simulink model "run_2022"  (R2022b)
settings: Solver=VariableStepAuto  StartTime=t_i  StopTime=2  MaxStep=s_max  RelTol=1e-3
InitFcn:
  | data;
  | init;
values from neighbouring files (symbols this model uses):
  h_ej = 0.15    [data.m]
  phi_0 = atan(-(r_ej*h_0)/(h_ej^2*sqrt(1-h_0^2/h_ej^2)))    [init.m]
  r_0 = sqrt((r_ej^2)*(1-h_0^2/h_ej^2))    [init.m]
  r_ej = 0.0821    [data.m]
  T_d = 1e-20    [data.m]
  x_ej = -0.05    [data.m]
  y_ej = 0.06    [data.m]
  z_ej = -0.03    [data.m]
undefined symbols (not defined in the file or in its folder): Glenohumeral_F0M, Glenohumeral_l0, Scapulothoracic_F0M, Scapulothoracic_l0, X, Y, Z
libraries: sm_lib x148, nesl_utility x62
(part 4 of 4)

== system run_2022/Scapulothoracic/TRP3 ==
  Aktivace : Inport
  Active_factor_norm : MATLAB Function  TreatAsAtomicUnit=on
  F0M : Gain  Gain=Scapulothoracic_F0M(7)
  Internal Force1 : sm_lib/Forces and Torques/Internal Force
  PECM1_3 : sm_lib/Frames and Transforms/Rigid Transform  TranslationMethod=Cartesian  TranslationStandardOffset=0  TranslationStandardOffsetUnits=m  TranslationStandardAxis=+Z  TranslationCartesianOffset=[-0.092 -0.015 0.003]  TranslationCartesianOffsetUnits=m  TranslationROffset=0  TranslationROffsetUnits=m  TranslationZOffset=0  TranslationZOffsetUnits=m  TranslationThetaOffset=0  TranslationThetaOffsetUnits=deg  RotationMethod=None  RotationAngleUnits=deg  RotationStandardAxis=+Z  RotationAngle=0.0  RotationArbitraryAxis=[0 0 1]  FollAlignAxisA=+X  BaseAlignAxisA=+Y  FollAlignAxisB=+Y  BaseAlignAxisB=+Z  RotationSequenceAxes=FollowerAxes  RotationSequence=XYX  RotationSequenceAngles=[0 0 0]  RotationSequenceAnglesUnits=deg  RotationMatrix=[1 0 0; 0 1 0; 0 0 1]  Quaternion=[1 0 0 0]
  PECM1_4 : sm_lib/Frames and Transforms/Rigid Transform  TranslationMethod=Cartesian  TranslationStandardOffset=0  TranslationStandardOffsetUnits=m  TranslationStandardAxis=+Z  TranslationCartesianOffset=[-0.058 -0.007 -0.044]  TranslationCartesianOffsetUnits=m  TranslationROffset=0  TranslationROffsetUnits=m  TranslationZOffset=0  TranslationZOffsetUnits=m  TranslationThetaOffset=0  TranslationThetaOffsetUnits=deg  RotationMethod=None  RotationAngleUnits=deg  RotationStandardAxis=+Y  RotationAngle=90  RotationArbitraryAxis=[0 0 1]  FollAlignAxisA=+X  BaseAlignAxisA=+Y  FollAlignAxisB=+Y  BaseAlignAxisB=+Z  RotationSequenceAxes=FollowerAxes  RotationSequence=XYX  RotationSequenceAngles=[0 0 0]  RotationSequenceAnglesUnits=deg  RotationMatrix=[1 0 0; 0 1 0; 0 0 1]  Quaternion=[1 0 0 0]
  PS-Simulink Converter : nesl_utility/PS-Simulink Converter  PhysicalDomain=network_engine_domain  SubClassName=ps_output  LeftPortType=input  RightPortType=output  PseudoPeriodic=off  Frequencies=[]  VectorFormat=inherit  Unit=inherit  AffineConversion=off
  Passive_force_norm : MATLAB Function  TreatAsAtomicUnit=on
  Simulink-PS Converter : nesl_utility/Simulink-PS Converter  PhysicalDomain=network_engine_domain  SubClassName=ps_input  LeftPortType=input  RightPortType=output  PseudoPeriodic=off  Frequencies=[]  NoiseDistribution=none  NoiseParameters=[]  Unit=1  AffineConversion=off  FilteringAndDerivatives=provide  SimscapeFilterOrder=1  InputFilterTimeConstant=0.001  UdotUserProvided=0
  Sum : Sum  Inputs=|++
  Tlak->Tah : Gain  Gain=-1
  Transform Sensor : sm_lib/Frames and Transforms/Transform Sensor  MeasurementFrame=World  RotationSequence=XYX  SenseAngle=off  SenseAxis=off  SenseQ=off  SenseR=off  SenseRotationSequence=off  SenseOmegaX=off  SenseOmegaY=off  SenseOmegaZ=off  SenseQDot=off  SenseRDot=off  SenseRotationSequenceDot=off  SenseAlphaX=off  SenseAlphaY=off  SenseAlphaZ=off  SenseQDDot=off  SenseRDDot=off  SenseX=off  SenseY=off  SenseZ=off  SenseRad=off  SenseAzim=off  SenseDist=on  SenseInc=off  SenseXDot=off  SenseYDot=off  SenseZDot=off  SenseRadDot=off  SenseAzimDot=off  SenseDistDot=off  SenseIncDot=off  SenseXDDot=off  SenseYDDot=off  SenseZDDot=off  SenseRadDDot=off  SenseAzimDDot=off  SenseDistDDot=off  SenseIncDDot=off
  l0m : Constant  Value=Scapulothoracic_l0(7)
  Thorax : PMIOPort  Side=Left
  Scapula : PMIOPort  Port=2  Side=Left
  Output : Outport
  Outport : Outport  Port=2
  wires:
  Aktivace/1 -> Active_factor_norm/3(a)
  PS-Simulink Converter/1 -> Outport/1, Active_factor_norm/1(lm), Passive_force_norm/1(lm)
  Active_factor_norm/1(Fa_norm) -> Sum/2
  l0m/1 -> Active_factor_norm/2(l0), Passive_force_norm/2(l0)
  Passive_force_norm/1(Fp_norm) -> Sum/1
  F0M/1 -> Tlak->Tah/1
  Tlak->Tah/1 -> Output/1, Simulink-PS Converter/1
  Sum/1 -> F0M/1
  connections:
  PECM1_4/RConn1 -- Internal Force1/LConn1 -- Transform Sensor/LConn1
  PECM1_3/RConn1 -- Internal Force1/RConn1 -- Transform Sensor/RConn1
  Transform Sensor/RConn2 -- PS-Simulink Converter/LConn1
  Simulink-PS Converter/RConn1 -- Internal Force1/LConn2
  PECM1_3/LConn1 -- Thorax/RConn1
  PECM1_4/LConn1 -- Scapula/RConn1

== system run_2022/Scapulothoracic/TRP4 ==
  Aktivace : Inport
  Active_factor_norm : MATLAB Function  TreatAsAtomicUnit=on
  F0M : Gain  Gain=Scapulothoracic_F0M(8)
  Internal Force1 : sm_lib/Forces and Torques/Internal Force
  PECM1_3 : sm_lib/Frames and Transforms/Rigid Transform  TranslationMethod=Cartesian  TranslationStandardOffset=0  TranslationStandardOffsetUnits=m  TranslationStandardAxis=+Z  TranslationCartesianOffset=[-0.116 -0.106 0.001]  TranslationCartesianOffsetUnits=m  TranslationROffset=0  TranslationROffsetUnits=m  TranslationZOffset=0  TranslationZOffsetUnits=m  TranslationThetaOffset=0  TranslationThetaOffsetUnits=deg  RotationMethod=None  RotationAngleUnits=deg  RotationStandardAxis=+Z  RotationAngle=0.0  RotationArbitraryAxis=[0 0 1]  FollAlignAxisA=+X  BaseAlignAxisA=+Y  FollAlignAxisB=+Y  BaseAlignAxisB=+Z  RotationSequenceAxes=FollowerAxes  RotationSequence=XYX  RotationSequenceAngles=[0 0 0]  RotationSequenceAnglesUnits=deg  RotationMatrix=[1 0 0; 0 1 0; 0 0 1]  Quaternion=[1 0 0 0]
  PECM1_4 : sm_lib/Frames and Transforms/Rigid Transform  TranslationMethod=Cartesian  TranslationStandardOffset=0  TranslationStandardOffsetUnits=m  TranslationStandardAxis=+Z  TranslationCartesianOffset=[-0.079 -0.013 -0.079]  TranslationCartesianOffsetUnits=m  TranslationROffset=0  TranslationROffsetUnits=m  TranslationZOffset=0  TranslationZOffsetUnits=m  TranslationThetaOffset=0  TranslationThetaOffsetUnits=deg  RotationMethod=None  RotationAngleUnits=deg  RotationStandardAxis=+Y  RotationAngle=90  RotationArbitraryAxis=[0 0 1]  FollAlignAxisA=+X  BaseAlignAxisA=+Y  FollAlignAxisB=+Y  BaseAlignAxisB=+Z  RotationSequenceAxes=FollowerAxes  RotationSequence=XYX  RotationSequenceAngles=[0 0 0]  RotationSequenceAnglesUnits=deg  RotationMatrix=[1 0 0; 0 1 0; 0 0 1]  Quaternion=[1 0 0 0]
  PS-Simulink Converter : nesl_utility/PS-Simulink Converter  PhysicalDomain=network_engine_domain  SubClassName=ps_output  LeftPortType=input  RightPortType=output  PseudoPeriodic=off  Frequencies=[]  VectorFormat=inherit  Unit=inherit  AffineConversion=off
  Passive_force_norm : MATLAB Function  TreatAsAtomicUnit=on
  Simulink-PS Converter : nesl_utility/Simulink-PS Converter  PhysicalDomain=network_engine_domain  SubClassName=ps_input  LeftPortType=input  RightPortType=output  PseudoPeriodic=off  Frequencies=[]  NoiseDistribution=none  NoiseParameters=[]  Unit=1  AffineConversion=off  FilteringAndDerivatives=provide  SimscapeFilterOrder=1  InputFilterTimeConstant=0.001  UdotUserProvided=0
  Sum : Sum  Inputs=|++
  Tlak->Tah : Gain  Gain=-1
  Transform Sensor : sm_lib/Frames and Transforms/Transform Sensor  MeasurementFrame=World  RotationSequence=XYX  SenseAngle=off  SenseAxis=off  SenseQ=off  SenseR=off  SenseRotationSequence=off  SenseOmegaX=off  SenseOmegaY=off  SenseOmegaZ=off  SenseQDot=off  SenseRDot=off  SenseRotationSequenceDot=off  SenseAlphaX=off  SenseAlphaY=off  SenseAlphaZ=off  SenseQDDot=off  SenseRDDot=off  SenseX=off  SenseY=off  SenseZ=off  SenseRad=off  SenseAzim=off  SenseDist=on  SenseInc=off  SenseXDot=off  SenseYDot=off  SenseZDot=off  SenseRadDot=off  SenseAzimDot=off  SenseDistDot=off  SenseIncDot=off  SenseXDDot=off  SenseYDDot=off  SenseZDDot=off  SenseRadDDot=off  SenseAzimDDot=off  SenseDistDDot=off  SenseIncDDot=off
  l0m : Constant  Value=Scapulothoracic_l0(8)
  Thorax : PMIOPort  Side=Left
  Scapula : PMIOPort  Port=2  Side=Left
  Output : Outport
  Outport : Outport  Port=2
  wires:
  Sum/1 -> F0M/1
  l0m/1 -> Active_factor_norm/2(l0), Passive_force_norm/2(l0)
  Passive_force_norm/1(Fp_norm) -> Sum/1
  Active_factor_norm/1(Fa_norm) -> Sum/2
  Aktivace/1 -> Active_factor_norm/3(a)
  F0M/1 -> Tlak->Tah/1
  Tlak->Tah/1 -> Output/1, Simulink-PS Converter/1
  PS-Simulink Converter/1 -> Active_factor_norm/1(lm), Passive_force_norm/1(lm), Outport/1
  connections:
  PECM1_4/RConn1 -- Internal Force1/LConn1 -- Transform Sensor/LConn1
  PECM1_3/RConn1 -- Internal Force1/RConn1 -- Transform Sensor/RConn1
  Simulink-PS Converter/RConn1 -- Internal Force1/LConn2
  PECM1_4/LConn1 -- Scapula/RConn1
  PECM1_3/LConn1 -- Thorax/RConn1
  Transform Sensor/RConn2 -- PS-Simulink Converter/LConn1

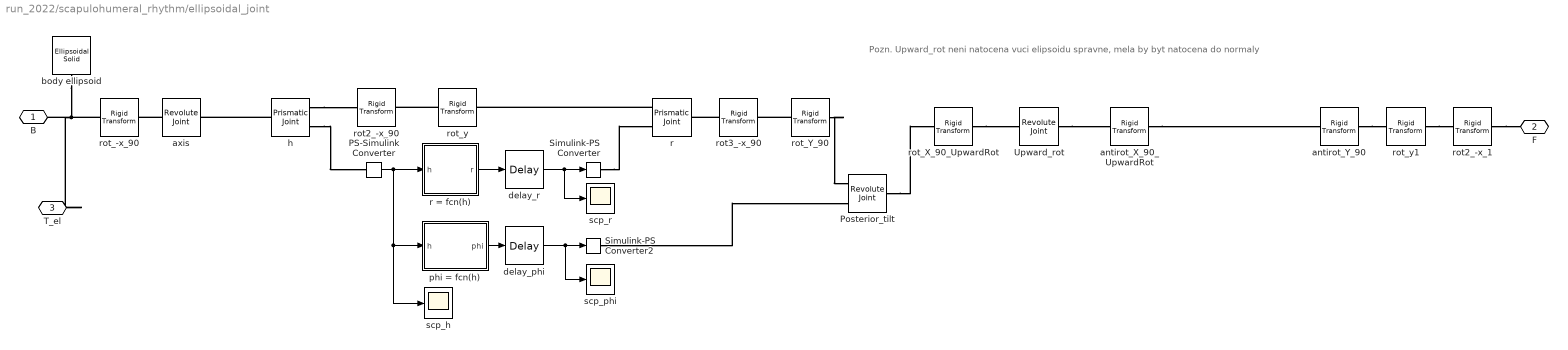
== system run_2022/scapulohumeral_rhythm/ellipsoidal_joint ==
  note: Pozn. Upward_rot neni natocena vuci elipsoidu spravne, mela by byt natocena do normaly
  PS-Simulink Converter : nesl_utility/PS-Simulink Converter  PhysicalDomain=network_engine_domain  SubClassName=ps_output  LeftPortType=input  RightPortType=output  PseudoPeriodic=off  Frequencies=[]  VectorFormat=inherit  Unit=inherit  AffineConversion=off
  Posterior_tilt : sm_lib/Joints/Revolute Joint  JointMode=Normal  SenseConstraintForce=off  SenseConstraintForceX=off  SenseConstraintForceY=off  SenseConstraintForceZ=off  SenseConstraintTorque=off  SenseConstraintTorqueX=off  SenseConstraintTorqueY=off  SenseConstraintTorqueZ=off  SenseTotalForce=off  SenseTotalForceX=off  SenseTotalForceY=off  SenseTotalForceZ=off  SenseTotalTorque=off  SenseTotalTorqueX=off  SenseTotalTorqueY=off  SenseTotalTorqueZ=off  CompositeWrenchDir=FollowerOnBase  CompositeWrenchFrame=BaseFrame  EquilibriumPosition=0  EquilibriumPositionUnits=deg  SpringStiffness=0  SpringStiffnessUnits=N*m/deg  DampingCoefficient=0  DampingCoefficientUnits=N*m/(deg/s)  TorqueActuationMode=ComputedTorque  MotionActuationMode=InputMotion  SensePosition=off  SenseVelocity=off  SenseAcceleration=off  SenseTorqueForce=off  SenseLowerLimitTorqueForce=off  SenseUpperLimitTorqueForce=off  LowerLimitSpecify=off  LowerLimitBound=-90  LowerLimitBoundUnits=deg  LowerLimitStiffness=1e4  LowerLimitStiffnessUnits=N*m/deg  LowerLimitDamping=10  LowerLimitDampingUnits=N*m/(deg/s)  LowerLimitTransitionRegionWidth=0.1  LowerLimitTransitionRegionWidthUnits=deg  UpperLimitSpecify=off  UpperLimitBound=90  UpperLimitBoundUnits=deg  UpperLimitStiffness=1e4  UpperLimitStiffnessUnits=N*m/deg  UpperLimitDamping=10  UpperLimitDampingUnits=N*m/(deg/s)  UpperLimitTransitionRegionWidth=0.1  UpperLimitTransitionRegionWidthUnits=deg  PositionTargetSpecify=on  PositionTargetPriority=High  PositionTargetValue=0  PositionTargetValueUnits=rad  VelocityTargetSpecify=off  VelocityTargetPriority=High  VelocityTargetValue=0  VelocityTargetValueUnits=deg/s
  Simulink-PS Converter : nesl_utility/Simulink-PS Converter  PhysicalDomain=network_engine_domain  SubClassName=ps_input  LeftPortType=input  RightPortType=output  PseudoPeriodic=off  Frequencies=[]  NoiseDistribution=none  NoiseParameters=[]  Unit=1  AffineConversion=off  FilteringAndDerivatives=filter  SimscapeFilterOrder=2  InputFilterTimeConstant=0.001  UdotUserProvided=0
  Simulink-PS Converter2 : nesl_utility/Simulink-PS Converter  PhysicalDomain=network_engine_domain  SubClassName=ps_input  LeftPortType=input  RightPortType=output  PseudoPeriodic=off  Frequencies=[]  NoiseDistribution=none  NoiseParameters=[]  Unit=1  AffineConversion=off  FilteringAndDerivatives=filter  SimscapeFilterOrder=2  InputFilterTimeConstant=0.001  UdotUserProvided=0
  Upward_rot : sm_lib/Joints/Revolute Joint  JointMode=Normal  SenseConstraintForce=off  SenseConstraintForceX=off  SenseConstraintForceY=off  SenseConstraintForceZ=off  SenseConstraintTorque=off  SenseConstraintTorqueX=off  SenseConstraintTorqueY=off  SenseConstraintTorqueZ=off  SenseTotalForce=off  SenseTotalForceX=off  SenseTotalForceY=off  SenseTotalForceZ=off  SenseTotalTorque=off  SenseTotalTorqueX=off  SenseTotalTorqueY=off  SenseTotalTorqueZ=off  CompositeWrenchDir=FollowerOnBase  CompositeWrenchFrame=BaseFrame  EquilibriumPosition=0  EquilibriumPositionUnits=deg  SpringStiffness=0  SpringStiffnessUnits=N*m/deg  DampingCoefficient=f_koef  DampingCoefficientUnits=N*m/(deg/s)  TorqueActuationMode=NoTorque  MotionActuationMode=ComputedMotion  SensePosition=off  SenseVelocity=off  SenseAcceleration=off  SenseTorqueForce=off  SenseLowerLimitTorqueForce=off  SenseUpperLimitTorqueForce=off  LowerLimitSpecify=off  LowerLimitBound=-90  LowerLimitBoundUnits=deg  LowerLimitStiffness=1e4  LowerLimitStiffnessUnits=N*m/deg  LowerLimitDamping=10  LowerLimitDampingUnits=N*m/(deg/s)  LowerLimitTransitionRegionWidth=0.1  LowerLimitTransitionRegionWidthUnits=deg  UpperLimitSpecify=off  UpperLimitBound=90  UpperLimitBoundUnits=deg  UpperLimitStiffness=1e4  UpperLimitStiffnessUnits=N*m/deg  UpperLimitDamping=10  UpperLimitDampingUnits=N*m/(deg/s)  UpperLimitTransitionRegionWidth=0.1  UpperLimitTransitionRegionWidthUnits=deg  PositionTargetSpecify=off  PositionTargetPriority=High  PositionTargetValue=0  PositionTargetValueUnits=deg  VelocityTargetSpecify=off  VelocityTargetPriority=High  VelocityTargetValue=0  VelocityTargetValueUnits=deg/s
  antirot_X_90_UpwardRot : sm_lib/Frames and Transforms/Rigid Transform  TranslationMethod=None  TranslationStandardOffset=0  TranslationStandardOffsetUnits=m  TranslationStandardAxis=+Z  TranslationCartesianOffset=[0 0 0]  TranslationCartesianOffsetUnits=m  TranslationROffset=0  TranslationROffsetUnits=m  TranslationZOffset=0  TranslationZOffsetUnits=m  TranslationThetaOffset=0  TranslationThetaOffsetUnits=deg  RotationMethod=StandardAxis  RotationAngleUnits=deg  RotationStandardAxis=+X  RotationAngle=-90  RotationArbitraryAxis=[0 0 1]  FollAlignAxisA=+X  BaseAlignAxisA=+Y  FollAlignAxisB=+Y  BaseAlignAxisB=+Z  RotationSequenceAxes=FollowerAxes  RotationSequence=XYX  RotationSequenceAngles=[0 0 0]  RotationSequenceAnglesUnits=deg  RotationMatrix=[1 0 0; 0 1 0; 0 0 1]  Quaternion=[1 0 0 0]
  antirot_Y_90 : sm_lib/Frames and Transforms/Rigid Transform  TranslationMethod=None  TranslationStandardOffset=0  TranslationStandardOffsetUnits=m  TranslationStandardAxis=+Z  TranslationCartesianOffset=[0 0 0]  TranslationCartesianOffsetUnits=m  TranslationROffset=0  TranslationROffsetUnits=m  TranslationZOffset=0  TranslationZOffsetUnits=m  TranslationThetaOffset=0  TranslationThetaOffsetUnits=deg  RotationMethod=StandardAxis  RotationAngleUnits=deg  RotationStandardAxis=+Y  RotationAngle=-90  RotationArbitraryAxis=[0 0 1]  FollAlignAxisA=+X  BaseAlignAxisA=+Y  FollAlignAxisB=+Y  BaseAlignAxisB=+Z  RotationSequenceAxes=FollowerAxes  RotationSequence=XYX  RotationSequenceAngles=[0 0 0]  RotationSequenceAnglesUnits=deg  RotationMatrix=[1 0 0; 0 1 0; 0 0 1]  Quaternion=[1 0 0 0]
  axis : sm_lib/Joints/Revolute Joint  JointMode=Normal  SenseConstraintForce=off  SenseConstraintForceX=off  SenseConstraintForceY=off  SenseConstraintForceZ=off  SenseConstraintTorque=off  SenseConstraintTorqueX=off  SenseConstraintTorqueY=off  SenseConstraintTorqueZ=off  SenseTotalForce=off  SenseTotalForceX=off  SenseTotalForceY=off  SenseTotalForceZ=off  SenseTotalTorque=off  SenseTotalTorqueX=off  SenseTotalTorqueY=off  SenseTotalTorqueZ=off  CompositeWrenchDir=FollowerOnBase  CompositeWrenchFrame=BaseFrame  EquilibriumPosition=0  EquilibriumPositionUnits=deg  SpringStiffness=0  SpringStiffnessUnits=N*m/deg  DampingCoefficient=f_koef  DampingCoefficientUnits=N*m/(deg/s)  TorqueActuationMode=NoTorque  MotionActuationMode=ComputedMotion  SensePosition=off  SenseVelocity=off  SenseAcceleration=off  SenseTorqueForce=off  SenseLowerLimitTorqueForce=off  SenseUpperLimitTorqueForce=off  LowerLimitSpecify=off  LowerLimitBound=-90  LowerLimitBoundUnits=deg  LowerLimitStiffness=1e4  LowerLimitStiffnessUnits=N*m/deg  LowerLimitDamping=10  LowerLimitDampingUnits=N*m/(deg/s)  LowerLimitTransitionRegionWidth=0.1  LowerLimitTransitionRegionWidthUnits=deg  UpperLimitSpecify=off  UpperLimitBound=90  UpperLimitBoundUnits=deg  UpperLimitStiffness=1e4  UpperLimitStiffnessUnits=N*m/deg  UpperLimitDamping=10  UpperLimitDampingUnits=N*m/(deg/s)  UpperLimitTransitionRegionWidth=0.1  UpperLimitTransitionRegionWidthUnits=deg  PositionTargetSpecify=off  PositionTargetPriority=High  PositionTargetValue=0  PositionTargetValueUnits=deg  VelocityTargetSpecify=off  VelocityTargetPriority=High  VelocityTargetValue=0  VelocityTargetValueUnits=deg/s
  body ellipsoid : sm_lib/Body Elements/Ellipsoidal Solid  GraphicAmbientColor=[0.15 0.15 0.15 1.0]  BasedOnType=Density  CenterOfMass=[0 0 0]  CenterOfMassUnits=m  GraphicDiffuseColor=[1 0 0]  Density=1000  DensityUnits=kg/m^3  DoExposeReferenceFrame=on  EllipsoidRadii="[r_ej h_ej  r_ej]"  EllipsoidRadiiUnits=m  GraphicEmissiveColor=[0.0 0.0 0.0 1.0]  ExportEntireGeometry=off  SerializedFrames=<Frames/>  MarkerShape=Sphere  MarkerSize=10  GraphicType=FromGeometry  InertiaType=PointMass  Mass=0.001  MassUnits=kg  MomentsOfInertia=[1 1 1]  MomentsOfInertiaUnits=kg*m^2  GraphicOpacity=0.2  ProductsOfInertia=[0 0 0]  ProductsOfInertiaUnits=kg*m^2  GraphicShininess=75  GraphicSpecularColor=[0.5 0.5 0.5 1.0]  GraphicVisPropType=SimpleVisualProperties
  delay_phi : TransportDelay  DelayTime=T_d
  delay_r : TransportDelay  DelayTime=T_d  InitialOutput=r_0
  h : sm_lib/Joints/Prismatic Joint  JointMode=Normal  SenseConstraintForce=off  SenseConstraintForceX=off  SenseConstraintForceY=off  SenseConstraintForceZ=off  SenseConstraintTorque=off  SenseConstraintTorqueX=off  SenseConstraintTorqueY=off  SenseConstraintTorqueZ=off  SenseTotalForce=off  SenseTotalForceX=off  SenseTotalForceY=off  SenseTotalForceZ=off  SenseTotalTorque=off  SenseTotalTorqueX=off  SenseTotalTorqueY=off  SenseTotalTorqueZ=off  CompositeWrenchDir=FollowerOnBase  CompositeWrenchFrame=BaseFrame  EquilibriumPosition=0  EquilibriumPositionUnits=m  SpringStiffness=0  SpringStiffnessUnits=N/m  DampingCoefficient=f_koef  DampingCoefficientUnits=N/(m/s)  TorqueActuationMode=NoTorque  MotionActuationMode=ComputedMotion  SensePosition=on  SenseVelocity=off  SenseAcceleration=off  SenseTorqueForce=off  SenseLowerLimitTorqueForce=off  SenseUpperLimitTorqueForce=off  LowerLimitSpecify=on  LowerLimitBound=h_min  LowerLimitBoundUnits=m  LowerLimitStiffness=1e6  LowerLimitStiffnessUnits=N/m  LowerLimitDamping=1e3  LowerLimitDampingUnits=N/(m/s)  LowerLimitTransitionRegionWidth=1e-4  LowerLimitTransitionRegionWidthUnits=m  UpperLimitSpecify=on  UpperLimitBound=h_max  UpperLimitBoundUnits=m  UpperLimitStiffness=1e6  UpperLimitStiffnessUnits=N/m  UpperLimitDamping=1e3  UpperLimitDampingUnits=N/(m/s)  UpperLimitTransitionRegionWidth=1e-4  UpperLimitTransitionRegionWidthUnits=m  PositionTargetSpecify=on  PositionTargetPriority=High  PositionTargetValue=h_0  PositionTargetValueUnits=m  VelocityTargetSpecify=off  VelocityTargetPriority=High  VelocityTargetValue=0  VelocityTargetValueUnits=m/s
  phi = fcn(h) : MATLAB Function  TreatAsAtomicUnit=on
  r : sm_lib/Joints/Prismatic Joint  JointMode=Normal  SenseConstraintForce=off  SenseConstraintForceX=off  SenseConstraintForceY=off  SenseConstraintForceZ=off  SenseConstraintTorque=off  SenseConstraintTorqueX=off  SenseConstraintTorqueY=off  SenseConstraintTorqueZ=off  SenseTotalForce=off  SenseTotalForceX=off  SenseTotalForceY=off  SenseTotalForceZ=off  SenseTotalTorque=off  SenseTotalTorqueX=off  SenseTotalTorqueY=off  SenseTotalTorqueZ=off  CompositeWrenchDir=FollowerOnBase  CompositeWrenchFrame=BaseFrame  EquilibriumPosition=0  EquilibriumPositionUnits=m  SpringStiffness=0  SpringStiffnessUnits=N/m  DampingCoefficient=0  DampingCoefficientUnits=N/(m/s)  TorqueActuationMode=ComputedTorque  MotionActuationMode=InputMotion  SensePosition=off  SenseVelocity=off  SenseAcceleration=off  SenseTorqueForce=off  SenseLowerLimitTorqueForce=off  SenseUpperLimitTorqueForce=off  LowerLimitSpecify=off  LowerLimitBound=-1  LowerLimitBoundUnits=m  LowerLimitStiffness=1e6  LowerLimitStiffnessUnits=N/m  LowerLimitDamping=1e3  LowerLimitDampingUnits=N/(m/s)  LowerLimitTransitionRegionWidth=1e-4  LowerLimitTransitionRegionWidthUnits=m  UpperLimitSpecify=off  UpperLimitBound=1  UpperLimitBoundUnits=m  UpperLimitStiffness=1e6  UpperLimitStiffnessUnits=N/m  UpperLimitDamping=1e3  UpperLimitDampingUnits=N/(m/s)  UpperLimitTransitionRegionWidth=1e-4  UpperLimitTransitionRegionWidthUnits=m  PositionTargetSpecify=off  PositionTargetPriority=High  PositionTargetValue=r_0  PositionTargetValueUnits=m  VelocityTargetSpecify=off  VelocityTargetPriority=High  VelocityTargetValue=0  VelocityTargetValueUnits=m/s
  r = fcn(h) : MATLAB Function  TreatAsAtomicUnit=on
  rot2_-x_1 : sm_lib/Frames and Transforms/Rigid Transform  TranslationMethod=None  TranslationStandardOffset=0  TranslationStandardOffsetUnits=m  TranslationStandardAxis=+Z  TranslationCartesianOffset=[0 0 0]  TranslationCartesianOffsetUnits=m  TranslationROffset=0  TranslationROffsetUnits=m  TranslationZOffset=0  TranslationZOffsetUnits=m  TranslationThetaOffset=0  TranslationThetaOffsetUnits=deg  RotationMethod=StandardAxis  RotationAngleUnits=deg  RotationStandardAxis=-X  RotationAngle=90  RotationArbitraryAxis=[0 0 1]  FollAlignAxisA=+X  BaseAlignAxisA=+Y  FollAlignAxisB=+Y  BaseAlignAxisB=+Z  RotationSequenceAxes=FollowerAxes  RotationSequence=XYX  RotationSequenceAngles=[0 0 0]  RotationSequenceAnglesUnits=deg  RotationMatrix=[1 0 0; 0 1 0; 0 0 1]  Quaternion=[1 0 0 0]
  rot2_-x_90 : sm_lib/Frames and Transforms/Rigid Transform  TranslationMethod=None  TranslationStandardOffset=0  TranslationStandardOffsetUnits=m  TranslationStandardAxis=+Z  TranslationCartesianOffset=[0 0 0]  TranslationCartesianOffsetUnits=m  TranslationROffset=0  TranslationROffsetUnits=m  TranslationZOffset=0  TranslationZOffsetUnits=m  TranslationThetaOffset=0  TranslationThetaOffsetUnits=deg  RotationMethod=StandardAxis  RotationAngleUnits=deg  RotationStandardAxis=-X  RotationAngle=90  RotationArbitraryAxis=[0 0 1]  FollAlignAxisA=+X  BaseAlignAxisA=+Y  FollAlignAxisB=+Y  BaseAlignAxisB=+Z  RotationSequenceAxes=FollowerAxes  RotationSequence=XYX  RotationSequenceAngles=[0 0 0]  RotationSequenceAnglesUnits=deg  RotationMatrix=[1 0 0; 0 1 0; 0 0 1]  Quaternion=[1 0 0 0]
  rot3_-x_90 : sm_lib/Frames and Transforms/Rigid Transform  TranslationMethod=None  TranslationStandardOffset=0  TranslationStandardOffsetUnits=m  TranslationStandardAxis=+Z  TranslationCartesianOffset=[0 0 0]  TranslationCartesianOffsetUnits=m  TranslationROffset=0  TranslationROffsetUnits=m  TranslationZOffset=0  TranslationZOffsetUnits=m  TranslationThetaOffset=0  TranslationThetaOffsetUnits=deg  RotationMethod=StandardAxis  RotationAngleUnits=deg  RotationStandardAxis=-X  RotationAngle=90  RotationArbitraryAxis=[0 0 1]  FollAlignAxisA=+X  BaseAlignAxisA=+Y  FollAlignAxisB=+Y  BaseAlignAxisB=+Z  RotationSequenceAxes=FollowerAxes  RotationSequence=XYX  RotationSequenceAngles=[0 0 0]  RotationSequenceAnglesUnits=deg  RotationMatrix=[1 0 0; 0 1 0; 0 0 1]  Quaternion=[1 0 0 0]
  rot_-x_90 : sm_lib/Frames and Transforms/Rigid Transform  TranslationMethod=None  TranslationStandardOffset=0  TranslationStandardOffsetUnits=m  TranslationStandardAxis=+Z  TranslationCartesianOffset=[0 0 0]  TranslationCartesianOffsetUnits=m  TranslationROffset=0  TranslationROffsetUnits=m  TranslationZOffset=0  TranslationZOffsetUnits=m  TranslationThetaOffset=0  TranslationThetaOffsetUnits=deg  RotationMethod=StandardAxis  RotationAngleUnits=deg  RotationStandardAxis=-X  RotationAngle=90  RotationArbitraryAxis=[0 0 1]  FollAlignAxisA=+X  BaseAlignAxisA=+Y  FollAlignAxisB=+Y  BaseAlignAxisB=+Z  RotationSequenceAxes=FollowerAxes  RotationSequence=XYX  RotationSequenceAngles=[0 0 0]  RotationSequenceAnglesUnits=deg  RotationMatrix=[1 0 0; 0 1 0; 0 0 1]  Quaternion=[1 0 0 0]
  rot_X_90_UpwardRot : sm_lib/Frames and Transforms/Rigid Transform  TranslationMethod=None  TranslationStandardOffset=0  TranslationStandardOffsetUnits=m  TranslationStandardAxis=+Z  TranslationCartesianOffset=[0 0 0]  TranslationCartesianOffsetUnits=m  TranslationROffset=0  TranslationROffsetUnits=m  TranslationZOffset=0  TranslationZOffsetUnits=m  TranslationThetaOffset=0  TranslationThetaOffsetUnits=deg  RotationMethod=StandardAxis  RotationAngleUnits=deg  RotationStandardAxis=+X  RotationAngle=90  RotationArbitraryAxis=[0 0 1]  FollAlignAxisA=+X  BaseAlignAxisA=+Y  FollAlignAxisB=+Y  BaseAlignAxisB=+Z  RotationSequenceAxes=FollowerAxes  RotationSequence=XYX  RotationSequenceAngles=[0 0 0]  RotationSequenceAnglesUnits=deg  RotationMatrix=[1 0 0; 0 1 0; 0 0 1]  Quaternion=[1 0 0 0]
  rot_Y_90 : sm_lib/Frames and Transforms/Rigid Transform  TranslationMethod=None  TranslationStandardOffset=0  TranslationStandardOffsetUnits=m  TranslationStandardAxis=+Z  TranslationCartesianOffset=[0 0 0]  TranslationCartesianOffsetUnits=m  TranslationROffset=0  TranslationROffsetUnits=m  TranslationZOffset=0  TranslationZOffsetUnits=m  TranslationThetaOffset=0  TranslationThetaOffsetUnits=deg  RotationMethod=StandardAxis  RotationAngleUnits=deg  RotationStandardAxis=+Y  RotationAngle=90  RotationArbitraryAxis=[0 0 1]  FollAlignAxisA=+X  BaseAlignAxisA=+Y  FollAlignAxisB=+Y  BaseAlignAxisB=+Z  RotationSequenceAxes=FollowerAxes  RotationSequence=XYX  RotationSequenceAngles=[0 0 0]  RotationSequenceAnglesUnits=deg  RotationMatrix=[1 0 0; 0 1 0; 0 0 1]  Quaternion=[1 0 0 0]
  rot_y : sm_lib/Frames and Transforms/Rigid Transform  TranslationMethod=None  TranslationStandardOffset=0  TranslationStandardOffsetUnits=m  TranslationStandardAxis=+Z  TranslationCartesianOffset=[0 0 0]  TranslationCartesianOffsetUnits=m  TranslationROffset=0  TranslationROffsetUnits=m  TranslationZOffset=0  TranslationZOffsetUnits=m  TranslationThetaOffset=0  TranslationThetaOffsetUnits=deg  RotationMethod=StandardAxis  RotationAngleUnits=deg  RotationStandardAxis=-Y  RotationAngle=90-51.694  RotationArbitraryAxis=[0 0 1]  FollAlignAxisA=+X  BaseAlignAxisA=+Y  FollAlignAxisB=+Y  BaseAlignAxisB=+Z  RotationSequenceAxes=FollowerAxes  RotationSequence=XYX  RotationSequenceAngles=[0 0 0]  RotationSequenceAnglesUnits=deg  RotationMatrix=[1 0 0; 0 1 0; 0 0 1]  Quaternion=[1 0 0 0]
  rot_y1 : sm_lib/Frames and Transforms/Rigid Transform  TranslationMethod=None  TranslationStandardOffset=0  TranslationStandardOffsetUnits=m  TranslationStandardAxis=+Z  TranslationCartesianOffset=[0 0 0]  TranslationCartesianOffsetUnits=m  TranslationROffset=0  TranslationROffsetUnits=m  TranslationZOffset=0  TranslationZOffsetUnits=m  TranslationThetaOffset=0  TranslationThetaOffsetUnits=deg  RotationMethod=StandardAxis  RotationAngleUnits=deg  RotationStandardAxis=+Z  RotationAngle=90-51.694  RotationArbitraryAxis=[0 0 1]  FollAlignAxisA=+X  BaseAlignAxisA=+Y  FollAlignAxisB=+Y  BaseAlignAxisB=+Z  RotationSequenceAxes=FollowerAxes  RotationSequence=XYX  RotationSequenceAngles=[0 0 0]  RotationSequenceAnglesUnits=deg  RotationMatrix=[1 0 0; 0 1 0; 0 0 1]  Quaternion=[1 0 0 0]
  scp_h : Scope
  scp_phi : Scope
  scp_r : Scope
  B : PMIOPort  Side=Left
  F : PMIOPort  Port=2  Side=Right
  T_el : PMIOPort  Port=3  Side=Left
  wires:
  PS-Simulink Converter/1 -> r = fcn(h)/1(h), scp_h/1, phi = fcn(h)/1(h)
  delay_r/1 -> scp_r/1, Simulink-PS Converter/1
  delay_phi/1 -> Simulink-PS Converter2/1, scp_phi/1
  r = fcn(h)/1(r) -> delay_r/1
  phi = fcn(h)/1(phi) -> delay_phi/1
  connections:
  body ellipsoid/RConn1 -- rot_-x_90/LConn1 -- T_el/RConn1 -- B/RConn1
  axis/LConn1 -- rot_-x_90/RConn1
  h/RConn2 -- PS-Simulink Converter/LConn1
  Simulink-PS Converter/RConn1 -- r/LConn2
  r/LConn1 -- rot_y/RConn1
  rot3_-x_90/LConn1 -- r/RConn1
  h/RConn1 -- rot2_-x_90/LConn1
  rot_y/LConn1 -- rot2_-x_90/RConn1
  h/LConn1 -- axis/RConn1
  rot_y1/RConn1 -- rot2_-x_1/LConn1
  rot2_-x_1/RConn1 -- F/RConn1
  antirot_Y_90/RConn1 -- rot_y1/LConn1
  rot_Y_90/LConn1 -- rot3_-x_90/RConn1
  rot_Y_90/RConn1 -- Posterior_tilt/LConn1
  Posterior_tilt/RConn1 -- rot_X_90_UpwardRot/LConn1
  Simulink-PS Converter2/RConn1 -- Posterior_tilt/LConn2
  rot_X_90_UpwardRot/RConn1 -- Upward_rot/LConn1
  antirot_X_90_UpwardRot/RConn1 -- antirot_Y_90/LConn1
  Upward_rot/RConn1 -- antirot_X_90_UpwardRot/LConn1

== matlab function run_2022/scapulohumeral_rhythm/ellipsoidal_joint/phi = fcn(h) ==
  data: h input; phi output; h_ej parameter; r_ej parameter; phi_0 parameter
function phi = fcn(h,h_ej,r_ej,phi_0)

phi = phi_0-atan(-(r_ej*h)/(h_ej^2*sqrt(1-h^2/h_ej^2)));

== matlab function run_2022/Glenohumeral/LAT/Passive_force_norm ==
  data: lm input; Fp_norm output; l0 input
function Fp_norm = fcn(lm,l0)
Fp_norm = ((lm/l0)^3)*exp(8*lm/l0-12.9);

== matlab function run_2022/Glenohumeral/PECM1/Active_factor_norm ==
  data: Fa_norm output; lm input; l0 input; a input
function Fa_norm = fcn(lm,l0,a)
f_gauss = 0.25;
Fa_norm = (exp(-(lm/l0-1)^2/f_gauss))*a;

== matlab function run_2022/Glenohumeral/PECM1/Passive_force_norm ==
  data: lm input; Fp_norm output; l0 input
function Fp_norm = fcn(lm,l0)
Fp_norm = ((lm/l0)^3)*exp(8*lm/l0-12.9);

== matlab function run_2022/Glenohumeral/PECM2/Active_factor_norm ==
  data: Fa_norm output; lm input; l0 input; a input
function Fa_norm = fcn(lm,l0,a)
f_gauss = 0.25;
Fa_norm = (exp(-(lm/l0-1)^2/f_gauss))*a;

== matlab function run_2022/Glenohumeral/PECM2/Passive_force_norm ==
  data: lm input; Fp_norm output; l0 input
function Fp_norm = fcn(lm,l0)
Fp_norm = ((lm/l0)^3)*exp(8*lm/l0-12.9);

== matlab function run_2022/Glenohumeral/PECM3/Active_factor_norm ==
  data: Fa_norm output; lm input; l0 input; a input
function Fa_norm = fcn(lm,l0,a)
f_gauss = 0.25;
Fa_norm = (exp(-(lm/l0-1)^2/f_gauss))*a;

== matlab function run_2022/Glenohumeral/PECM3/Passive_force_norm ==
  data: lm input; Fp_norm output; l0 input
function Fp_norm = fcn(lm,l0)
Fp_norm = ((lm/l0)^3)*exp(8*lm/l0-12.9);

== matlab function run_2022/Glenohumeral/SUBSC/Active_factor_norm ==
  data: Fa_norm output; lm input; l0 input; a input
function Fa_norm = fcn(lm,l0,a)
f_gauss = 0.25;
Fa_norm = (exp(-(lm/l0-1)^2/f_gauss))*a;

== matlab function run_2022/Glenohumeral/SUBSC/Passive_force_norm ==
  data: lm input; Fp_norm output; l0 input
function Fp_norm = fcn(lm,l0)
Fp_norm = ((lm/l0)^3)*exp(8*lm/l0-12.9);

== matlab function run_2022/Glenohumeral/SUPSP/Active_factor_norm ==
  data: Fa_norm output; lm input; l0 input; a input
function Fa_norm = fcn(lm,l0,a)
f_gauss = 0.25;
Fa_norm = (exp(-(lm/l0-1)^2/f_gauss))*a;

== matlab function run_2022/Glenohumeral/SUPSP/Passive_force_norm ==
  data: lm input; Fp_norm output; l0 input
function Fp_norm = fcn(lm,l0)
Fp_norm = ((lm/l0)^3)*exp(8*lm/l0-12.9);

== matlab function run_2022/Glenohumeral/TMAJ/Active_factor_norm ==
  data: Fa_norm output; lm input; l0 input; a input
function Fa_norm = fcn(lm,l0,a)
f_gauss = 0.25;
Fa_norm = (exp(-(lm/l0-1)^2/f_gauss))*a;

== matlab function run_2022/scapulohumeral_rhythm/ellipsoidal_joint/r = fcn(h) ==
  data: h input; r output; h_ej parameter; r_ej parameter
function r = fcn(h,h_ej,r_ej)

r = sqrt((r_ej^2)*(1-h^2/h_ej^2));

== matlab function run_2022/Glenohumeral/TMAJ/Passive_force_norm ==
  data: lm input; Fp_norm output; l0 input
function Fp_norm = fcn(lm,l0)
Fp_norm = ((lm/l0)^3)*exp(8*lm/l0-12.9);

== matlab function run_2022/Glenohumeral/TMIN/Active_factor_norm ==
  data: Fa_norm output; lm input; l0 input; a input
function Fa_norm = fcn(lm,l0,a)
f_gauss = 0.25;
Fa_norm = (exp(-(lm/l0-1)^2/f_gauss))*a;

== matlab function run_2022/Glenohumeral/TMIN/Passive_force_norm ==
  data: lm input; Fp_norm output; l0 input
function Fp_norm = fcn(lm,l0)
Fp_norm = ((lm/l0)^3)*exp(8*lm/l0-12.9);

== matlab function run_2022/Glenohumeral/CORB/Active_factor_norm ==
  data: Fa_norm output; lm input; l0 input; a input
function Fa_norm = fcn(lm,l0,a)
f_gauss = 0.25;
Fa_norm = (exp(-(lm/l0-1)^2/f_gauss))*a;

== matlab function run_2022/Glenohumeral/CORB/Passive_force_norm ==
  data: lm input; Fp_norm output; l0 input
function Fp_norm = fcn(lm,l0)
Fp_norm = ((lm/l0)^3)*exp(8*lm/l0-12.9);

== matlab function run_2022/Scapulothoracic/SBCL/Active_factor_norm ==
  data: Fa_norm output; lm input; l0 input; a input
function Fa_norm = fcn(lm,l0,a)
f_gauss = 0.25;
Fa_norm = (exp(-(lm/l0-1)^2/f_gauss))*a;

== matlab function run_2022/Scapulothoracic/SBCL/Passive_force_norm ==
  data: lm input; Fp_norm output; l0 input
function Fp_norm = fcn(lm,l0)
Fp_norm = ((lm/l0)^3)*exp(8*lm/l0-12.9);

== matlab function run_2022/Scapulothoracic/SRA1/Active_factor_norm ==
  data: Fa_norm output; lm input; l0 input; a input
function Fa_norm = fcn(lm,l0,a)
f_gauss = 0.25;
Fa_norm = (exp(-(lm/l0-1)^2/f_gauss))*a;

== matlab function run_2022/Scapulothoracic/SRA1/Passive_force_norm ==
  data: lm input; Fp_norm output; l0 input
function Fp_norm = fcn(lm,l0)
Fp_norm = ((lm/l0)^3)*exp(8*lm/l0-12.9);

== matlab function run_2022/Scapulothoracic/SRA2/Active_factor_norm ==
  data: Fa_norm output; lm input; l0 input; a input
function Fa_norm = fcn(lm,l0,a)
f_gauss = 0.25;
Fa_norm = (exp(-(lm/l0-1)^2/f_gauss))*a;

== matlab function run_2022/Glenohumeral/DELT1/Passive_force_norm ==
  data: lm input; Fp_norm output; l0 input
function Fp_norm = fcn(lm,l0)
Fp_norm = ((lm/l0)^3)*exp(8*lm/l0-12.9);

== matlab function run_2022/Scapulothoracic/SRA2/Passive_force_norm ==
  data: lm input; Fp_norm output; l0 input
function Fp_norm = fcn(lm,l0)
Fp_norm = ((lm/l0)^3)*exp(8*lm/l0-12.9);

== matlab function run_2022/Scapulothoracic/SRA3/Active_factor_norm ==
  data: Fa_norm output; lm input; l0 input; a input
function Fa_norm = fcn(lm,l0,a)
f_gauss = 0.25;
Fa_norm = (exp(-(lm/l0-1)^2/f_gauss))*a;

== matlab function run_2022/Scapulothoracic/SRA3/Passive_force_norm ==
  data: lm input; Fp_norm output; l0 input
function Fp_norm = fcn(lm,l0)
Fp_norm = ((lm/l0)^3)*exp(8*lm/l0-12.9);

== matlab function run_2022/Scapulothoracic/TRP1/Active_factor_norm ==
  data: Fa_norm output; lm input; l0 input; a input
function Fa_norm = fcn(lm,l0,a)
f_gauss = 0.25;
Fa_norm = (exp(-(lm/l0-1)^2/f_gauss))*a;

== matlab function run_2022/Scapulothoracic/TRP1/Passive_force_norm ==
  data: lm input; Fp_norm output; l0 input
function Fp_norm = fcn(lm,l0)
Fp_norm = ((lm/l0)^3)*exp(8*lm/l0-12.9);

== matlab function run_2022/Scapulothoracic/TRP2/Active_factor_norm ==
  data: Fa_norm output; lm input; l0 input; a input
function Fa_norm = fcn(lm,l0,a)
f_gauss = 0.25;
Fa_norm = (exp(-(lm/l0-1)^2/f_gauss))*a;

== matlab function run_2022/Scapulothoracic/TRP2/Passive_force_norm ==
  data: lm input; Fp_norm output; l0 input
function Fp_norm = fcn(lm,l0)
Fp_norm = ((lm/l0)^3)*exp(8*lm/l0-12.9);

== matlab function run_2022/Scapulothoracic/TRP3/Active_factor_norm ==
  data: Fa_norm output; lm input; l0 input; a input
function Fa_norm = fcn(lm,l0,a)
f_gauss = 0.25;
Fa_norm = (exp(-(lm/l0-1)^2/f_gauss))*a;

== matlab function run_2022/Scapulothoracic/TRP3/Passive_force_norm ==
  data: lm input; Fp_norm output; l0 input
function Fp_norm = fcn(lm,l0)
Fp_norm = ((lm/l0)^3)*exp(8*lm/l0-12.9);

== matlab function run_2022/Scapulothoracic/TRP4/Active_factor_norm ==
  data: Fa_norm output; lm input; l0 input; a input
function Fa_norm = fcn(lm,l0,a)
f_gauss = 0.25;
Fa_norm = (exp(-(lm/l0-1)^2/f_gauss))*a;

== matlab function run_2022/Glenohumeral/DELT1/Active_factor_norm ==
  data: Fa_norm output; lm input; l0 input; a input
function Fa_norm = fcn(lm,l0,a)
f_gauss = 0.25;
Fa_norm = (exp(-(lm/l0-1)^2/f_gauss))*a;

== matlab function run_2022/Scapulothoracic/TRP4/Passive_force_norm ==
  data: lm input; Fp_norm output; l0 input
function Fp_norm = fcn(lm,l0)
Fp_norm = ((lm/l0)^3)*exp(8*lm/l0-12.9);

== matlab function run_2022/Scapulothoracic/LVS/Active_factor_norm ==
  data: Fa_norm output; lm input; l0 input; a input
function Fa_norm = fcn(lm,l0,a)
f_gauss = 0.25;
Fa_norm = (exp(-(lm/l0-1)^2/f_gauss))*a;

== matlab function run_2022/Scapulothoracic/LVS/Passive_force_norm ==
  data: lm input; Fp_norm output; l0 input
function Fp_norm = fcn(lm,l0)
Fp_norm = ((lm/l0)^3)*exp(8*lm/l0-12.9);

== matlab function run_2022/Scapulothoracic/RMN/Active_factor_norm ==
  data: Fa_norm output; lm input; l0 input; a input
function Fa_norm = fcn(lm,l0,a)
f_gauss = 0.25;
Fa_norm = (exp(-(lm/l0-1)^2/f_gauss))*a;

== matlab function run_2022/Scapulothoracic/RMN/Passive_force_norm ==
  data: lm input; Fp_norm output; l0 input
function Fp_norm = fcn(lm,l0)
Fp_norm = ((lm/l0)^3)*exp(8*lm/l0-12.9);

== matlab function run_2022/Scapulothoracic/RMNJ1/Active_factor_norm ==
  data: Fa_norm output; lm input; l0 input; a input
function Fa_norm = fcn(lm,l0,a)
f_gauss = 0.25;
Fa_norm = (exp(-(lm/l0-1)^2/f_gauss))*a;

== matlab function run_2022/Scapulothoracic/RMNJ1/Passive_force_norm ==
  data: lm input; Fp_norm output; l0 input
function Fp_norm = fcn(lm,l0)
Fp_norm = ((lm/l0)^3)*exp(8*lm/l0-12.9);

== matlab function run_2022/Scapulothoracic/RMNJ2/Active_factor_norm ==
  data: Fa_norm output; lm input; l0 input; a input
function Fa_norm = fcn(lm,l0,a)
f_gauss = 0.25;
Fa_norm = (exp(-(lm/l0-1)^2/f_gauss))*a;

== matlab function run_2022/Scapulothoracic/RMNJ2/Passive_force_norm ==
  data: lm input; Fp_norm output; l0 input
function Fp_norm = fcn(lm,l0)
Fp_norm = ((lm/l0)^3)*exp(8*lm/l0-12.9);

== matlab function run_2022/Scapulothoracic/PMN/Active_factor_norm ==
  data: Fa_norm output; lm input; l0 input; a input
function Fa_norm = fcn(lm,l0,a)
f_gauss = 0.25;
Fa_norm = (exp(-(lm/l0-1)^2/f_gauss))*a;

== matlab function run_2022/Glenohumeral/DELT2/Active_factor_norm ==
  data: Fa_norm output; lm input; l0 input; a input
function Fa_norm = fcn(lm,l0,a)
f_gauss = 0.25;
Fa_norm = (exp(-(lm/l0-1)^2/f_gauss))*a;

== matlab function run_2022/Scapulothoracic/PMN/Passive_force_norm ==
  data: lm input; Fp_norm output; l0 input
function Fp_norm = fcn(lm,l0)
Fp_norm = ((lm/l0)^3)*exp(8*lm/l0-12.9);

== matlab function run_2022/Glenohumeral/DELT2/Passive_force_norm ==
  data: lm input; Fp_norm output; l0 input
function Fp_norm = fcn(lm,l0)
Fp_norm = ((lm/l0)^3)*exp(8*lm/l0-12.9);

== matlab function run_2022/Glenohumeral/DELT3/Active_factor_norm ==
  data: Fa_norm output; lm input; l0 input; a input
function Fa_norm = fcn(lm,l0,a)
f_gauss = 0.25;
Fa_norm = (exp(-(lm/l0-1)^2/f_gauss))*a;

== matlab function run_2022/Glenohumeral/DELT3/Passive_force_norm ==
  data: lm input; Fp_norm output; l0 input
function Fp_norm = fcn(lm,l0)
Fp_norm = ((lm/l0)^3)*exp(8*lm/l0-12.9);

== matlab function run_2022/Glenohumeral/INFRSP/Active_factor_norm ==
  data: Fa_norm output; lm input; l0 input; a input
function Fa_norm = fcn(lm,l0,a)
f_gauss = 0.25;
Fa_norm = (exp(-(lm/l0-1)^2/f_gauss))*a;

== matlab function run_2022/Glenohumeral/INFRSP/Passive_force_norm ==
  data: lm input; Fp_norm output; l0 input
function Fp_norm = fcn(lm,l0)
Fp_norm = ((lm/l0)^3)*exp(8*lm/l0-12.9);

== matlab function run_2022/Glenohumeral/LAT/Active_factor_norm ==
  data: Fa_norm output; lm input; l0 input; a input
function Fa_norm = fcn(lm,l0,a)
f_gauss = 0.25;
Fa_norm = (exp(-(lm/l0-1)^2/f_gauss))*a;
